simulink model "whirlybirdsim_trim"  (Simulink 7.5)
settings: Solver=ode45  StartTime=0.0  StopTime=100  RelTol=1e-3
values from neighbouring files (symbols this model uses):
  P = defineParameters    [plotWhirlybird.m]
settings Model: Creator=Administrator  LastModifiedBy=rwb5
settings DebuggingCC: StrictBusMsg=Warning

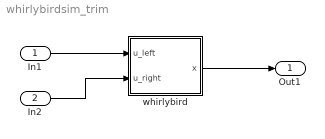
== system whirlybirdsim_trim ==
  In1 : Inport  OutDataType=fixdt(1, 16)  OutScaling=2^0
  In2 : Inport  Port=2  OutDataType=fixdt(1, 16)  OutScaling=2^0
  whirlybird : Subsystem
      mask Display: image(imread('whirlybird.jpg'))
  Out1 : Outport  OutDataType=fixdt(1, 16)  OutScaling=2^0
  wires:
  In1/1 -> whirlybird/1(u_left)
  In2/1 -> whirlybird/2(u_right)
  whirlybird/1(x) -> Out1/1

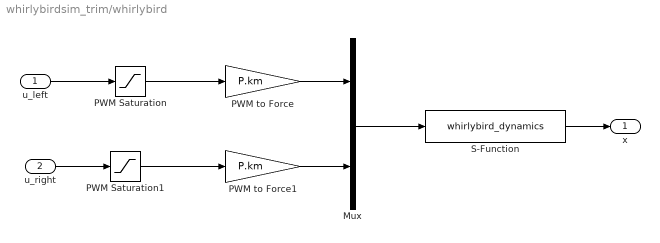
== system whirlybirdsim_trim/whirlybird ==
  u_left : Inport
  u_right : Inport  Port=2
  Mux : Mux  Inputs=2
  PWM Saturation : Saturate  UpperLimit=100  LowerLimit=0  OutDataType=sfix(16)  OutScaling=2^0
  PWM Saturation1 : Saturate  UpperLimit=100  LowerLimit=0  OutDataType=sfix(16)  OutScaling=2^0
  PWM to Force : Gain  Gain=P.km  ParameterDataType=sfix(16)  ParameterScaling=2^0  OutDataType=sfix(16)  OutScaling=2^0
  PWM to Force1 : Gain  Gain=P.km  ParameterDataType=sfix(16)  ParameterScaling=2^0  OutDataType=sfix(16)  OutScaling=2^0
  S-Function : S-Function  FunctionName=whirlybird_dynamics  Parameters=P  EnableBusSupport=off
  x : Outport
  wires:
  S-Function/1 -> x/1
  Mux/1 -> S-Function/1
  PWM to Force/1 -> Mux/1
  PWM Saturation/1 -> PWM to Force/1
  u_left/1 -> PWM Saturation/1
  u_right/1 -> PWM Saturation1/1
  PWM to Force1/1 -> Mux/2
  PWM Saturation1/1 -> PWM to Force1/1
